simulink model "WaitResponseTop"  (R2015a)
settings: Solver=FixedStepDiscrete  StartTime=0.0  StopTime=1.0  FixedStep=0.01  RelTol=1e-3
libraries: WaitResponse x1
settings Model: Creator=mbd_user  LastModifiedBy=mbd_user

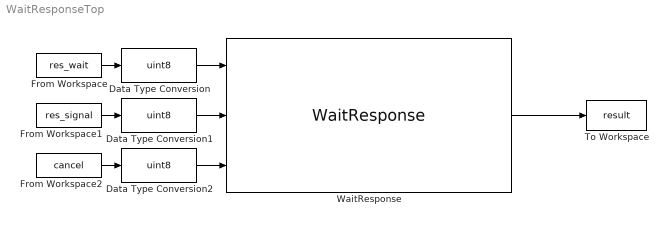
== system WaitResponseTop ==
  Data Type Conversion : DataTypeConversion  OutDataTypeStr=uint8  RndMeth=Nearest
  Data Type Conversion1 : DataTypeConversion  OutDataTypeStr=uint8  RndMeth=Nearest
  Data Type Conversion2 : DataTypeConversion  OutDataTypeStr=uint8  RndMeth=Nearest
  From Workspace : FromWorkspace  VariableName=res_wait  SampleTime=0
  From Workspace1 : FromWorkspace  VariableName=res_signal  SampleTime=0
  From Workspace2 : FromWorkspace  VariableName=cancel  SampleTime=0
  To Workspace : ToWorkspace  VariableName=result  SampleTime=-1
  WaitResponse : WaitResponse/WaitResponse
  wires:
  From Workspace/1 -> Data Type Conversion/1
  Data Type Conversion/1 -> WaitResponse/1
  From Workspace1/1 -> Data Type Conversion1/1
  Data Type Conversion1/1 -> WaitResponse/2
  From Workspace2/1 -> Data Type Conversion2/1
  Data Type Conversion2/1 -> WaitResponse/3
  WaitResponse/1 -> To Workspace/1
